simulink model "fw_pos_control"  (R2021a)
settings: Solver=FixedStepAuto  StartTime=0.0  StopTime=5  FixedStep=0.02  RelTol=1e-3
undefined symbols (not defined in the file): DiscIntNeverNeededParam, DT_DEFAULT, FW_AIRSPD_MAX, FW_AIRSPD_MIN, FW_L1_DAMPING, FW_L1_PERIOD, FW_L1_R_SLEW_MAX, FW_R_LIM, FW_T_CLMB_MAX, FW_T_HRATE_FF, FW_T_I_GAIN_PIT, FW_T_I_GAIN_THR, FW_T_PTCH_DAMP, FW_T_RLL2THR, FW_T_SEB_R_FF, FW_T_SINK_MAX, FW_T_SINK_MIN, FW_T_SPD_OMEGA, FW_T_STE_R_TC, FW_T_TAS_TC, FW_T_THR_DAMP, FW_T_VERT_ACC, FW_THR_CRUISE, FW_THR_MAX, FW_THR_MIN, FW_THR_SLEW_MAX, GRAVITY, magnitude
libraries: simulink x28, vrlib x3
(part 1 of 4)
settings Model: DataDictionary=px4_dict.sldd  Creator=DELL  LastModifiedBy=DELL
settings OptimizationCC: DefaultUnderspecifiedDataType=single
settings SFSimCC: SimTargetLang=C++

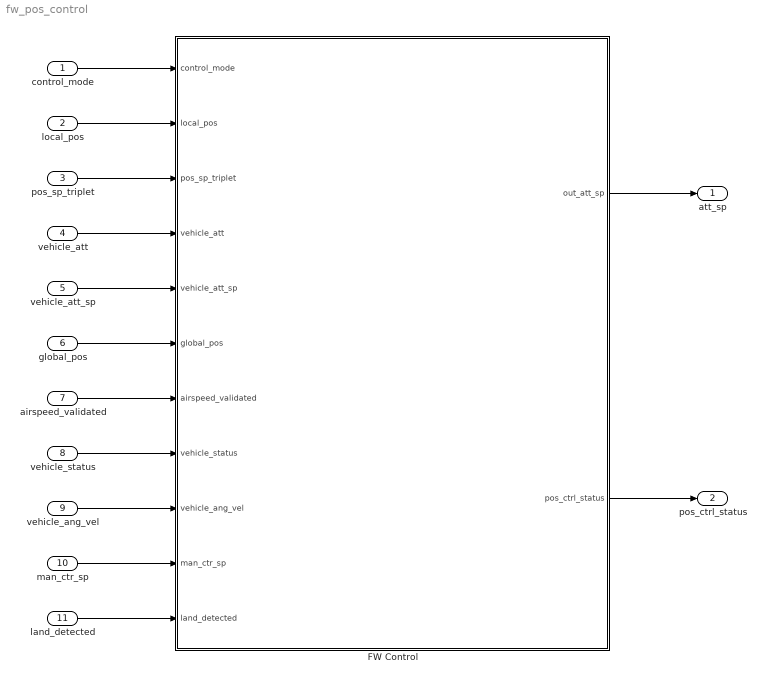
== system fw_pos_control ==
  control_mode : Inport  OutDataTypeStr=Bus: px4_vehicle_control_mode
  local_pos : Inport  Port=2  OutDataTypeStr=Bus: px4_vehicle_local_position
  pos_sp_triplet : Inport  Port=3  OutDataTypeStr=Bus: px4_position_setpoint_triplet
  vehicle_att : Inport  Port=4  OutDataTypeStr=Bus: px4_vehicle_attitude
  vehicle_att_sp : Inport  Port=5  OutDataTypeStr=Bus: px4_vehicle_attitude_setpoint
  global_pos : Inport  Port=6  OutDataTypeStr=Bus: px4_vehicle_global_position
  airspeed_validated : Inport  Port=7  OutDataTypeStr=Bus: px4_airspeed_validated
  vehicle_status : Inport  Port=8  OutDataTypeStr=Bus: px4_vehicle_status
  vehicle_ang_vel : Inport  Port=9  OutDataTypeStr=Bus: px4_vehicle_angular_velocity
  man_ctr_sp : Inport  Port=10  OutDataTypeStr=Bus: px4_manual_control_setpoint
  land_detected : Inport  Port=11  OutDataTypeStr=Bus: px4_vehicle_land_detected
  FW Control : Stateflow chart  TreatAsAtomicUnit=on
  att_sp : Outport
  pos_ctrl_status : Outport  Port=2
  wires:
  airspeed_validated/1 -> FW Control/7(airspeed_validated)
  vehicle_att/1 -> FW Control/4(vehicle_att)
  local_pos/1 -> FW Control/2(local_pos)
  man_ctr_sp/1 -> FW Control/10(man_ctr_sp)
  land_detected/1 -> FW Control/11(land_detected)
  vehicle_status/1 -> FW Control/8(vehicle_status)
  vehicle_att_sp/1 -> FW Control/5(vehicle_att_sp)
  control_mode/1 -> FW Control/1(control_mode)
  FW Control/1(out_att_sp) -> att_sp/1
  vehicle_ang_vel/1 -> FW Control/9(vehicle_ang_vel)
  global_pos/1 -> FW Control/6(global_pos)
  pos_sp_triplet/1 -> FW Control/3(pos_sp_triplet)
  FW Control/2(pos_ctrl_status) -> pos_ctrl_status/1

== system fw_pos_control/FW Control/fixed_wing.position_control.mode_action.l1_navigate_heading ==
  navigation_heading : Inport  OutDataTypeStr=single  PortDimensions=1
  current_heading : Inport  Port=2  OutDataTypeStr=single  PortDimensions=1
  ground_speed_vector : Inport  Port=3  OutDataTypeStr=single  PortDimensions=[1 2]
  att_sp_roll_body : Inport  Port=4  OutDataTypeStr=single  PortDimensions=1
  f : TriggerPort  TriggerType=function-call  VariantControl=(inherit)
      settings: CopyFcn=Stateflow.SLINSF.SimulinkMan.removeBlockPreDeleteFcn  PreDeleteFcn=Stateflow.SLINSF.SimulinkMan.unsafePredeleteFcn
  Constant : Constant  Value=sqrt(2) * pi / FW_L1_PERIOD
      settings: AttributesFormatString=%<Value>
  Constant1 : Constant  Value=false
  Divide : Product  Inputs=*/
  Dot Product1 : DotProduct  InputSameDT=on  OutDataTypeStr=Inherit: Inherit via internal rule
  Gain : Gain  Gain=sqrt(2) * pi / FW_L1_PERIOD
      settings: AttributesFormatString=%<Gain>
  Gain1 : Gain  Gain=2.0
  Product : Product
  Saturation1 : Saturate  UpperLimit=single(pi/2)  LowerLimit=single(-pi/2)
      settings: AttributesFormatString=[%<LowerLimit>,%<UpperLimit>]
  Sin : Trigonometry
  Sqrt1 : Sqrt  SaturateOnIntegerOverflow=on
  Sum : Sum  Inputs=|+-
  Update Roll Setpoint : Subsystem
  wrap -pi~pi : Subsystem
  roll_sp : Outport
  circle_mode : Outport  Port=2
  l1_heading_dis : Outport  Port=3
  wires:
  Constant1/1 -> circle_mode/1
  wrap -pi~pi/1(out) -> Saturation1/1  "eta"
  Sum/1 -> wrap -pi~pi/1(in)
  Saturation1/1 -> Sin/1
  navigation_heading/1 -> Sum/1
  current_heading/1 -> Sum/2
  Dot Product1/1 -> Sqrt1/1
  ground_speed_vector/1 -> Dot Product1/1, Dot Product1/2
  Sqrt1/1 -> Divide/1, Gain/1  "ground_speed_length"
  Product/1 -> Gain1/1
  Sin/1 -> Product/1
  Gain/1 -> Product/2
  Constant/1 -> Divide/2  "heading_omega"
  Divide/1 -> l1_heading_dis/1
  att_sp_roll_body/1 -> Update Roll Setpoint/1(att_sp_roll_body1)
  Gain1/1 -> Update Roll Setpoint/2(lateral_accel)
  Update Roll Setpoint/1(roll_new) -> roll_sp/1

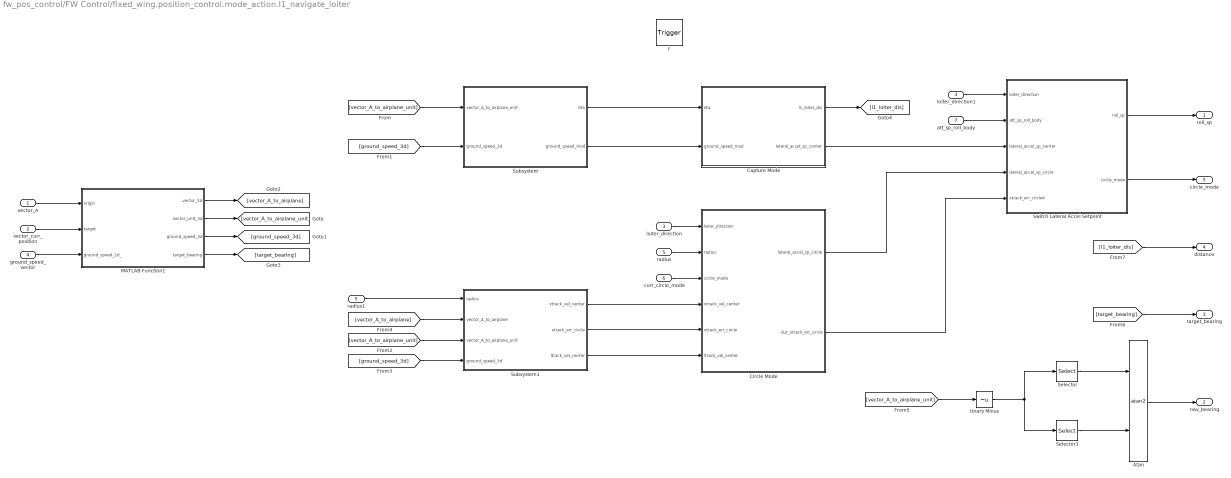
== system fw_pos_control/FW Control/fixed_wing.position_control.mode_action.l1_navigate_loiter ==
  vector_A : Inport  OutDataTypeStr=double  PortDimensions=[1 2]
  vector_curr_position : Inport  Port=2  OutDataTypeStr=double  PortDimensions=[1 2]
  loiter_direction : Inport  Port=3  OutDataTypeStr=int8  PortDimensions=1
  ground_speed_vector : Inport  Port=4  OutDataTypeStr=single  PortDimensions=[1 2]
  radius : Inport  Port=5  OutDataTypeStr=single  PortDimensions=1
  curr_circle_mode : Inport  Port=6  OutDataTypeStr=boolean  PortDimensions=1
  att_sp_roll_body : Inport  Port=7  OutDataTypeStr=single  PortDimensions=1
  f : TriggerPort  TriggerType=function-call  VariantControl=(inherit)
      settings: CopyFcn=Stateflow.SLINSF.SimulinkMan.removeBlockPreDeleteFcn  PreDeleteFcn=Stateflow.SLINSF.SimulinkMan.unsafePredeleteFcn
  Atan : Trigonometry  Operator=atan2
  Capture Mode : Subsystem
  Circle Mode : Subsystem
  MATLAB Function1 : MATLAB Function  TreatAsAtomicUnit=on
  Selector : Selector  InputPortWidth=3  IndexOptions=Index vector (dialog)  Indices=[2]  OutputSizes=1
  Selector1 : Selector  InputPortWidth=3  IndexOptions=Index vector (dialog)  Indices=[1]  OutputSizes=1
  Subsystem : Subsystem
  Subsystem1 : Subsystem
  Switch Lateral Accel Setpoint : Subsystem
  Unary Minus : UnaryMinus
  loiter_direction1 : InportShadow  Port=3  OutDataTypeStr=int8  PortDimensions=1
  radius1 : InportShadow  Port=5  OutDataTypeStr=single  PortDimensions=1
  roll_sp : Outport
  nav_bearing : Outport  Port=2
  target_bearing : Outport  Port=3
  distance : Outport  Port=4
  circle_mode : Outport  Port=5
  wires:
  vector_curr_position/1 -> MATLAB Function1/2(target)
  vector_A/1 -> MATLAB Function1/1(origin)
  ground_speed_vector/1 -> MATLAB Function1/3(ground_speed_2d_)
  Subsystem/1(eta) -> Capture Mode/1(eta)
  Capture Mode/2(lateral_accel_sp_center) -> Switch Lateral Accel Setpoint/3(lateral_accel_sp_center)
  Capture Mode/1(l1_loiter_dis) -> [l1_loiter_dis]
  Subsystem/2(ground_speed_mod) -> Capture Mode/2(ground_speed_mod)
  loiter_direction/1 -> Circle Mode/1(loiter_direction)
  radius/1 -> Circle Mode/2(radius)
  Circle Mode/1(lateral_accel_sp_circle) -> Switch Lateral Accel Setpoint/4(lateral_accel_sp_circle)
  Subsystem1/2(xtrack_err_circle) -> Circle Mode/5(xtrack_err_circle)
  Subsystem1/1(xtrack_vel_center) -> Circle Mode/4(xtrack_vel_center)
  MATLAB Function1/2(vector_unit_3d) -> [vector_A_to_airplane_unit]
  MATLAB Function1/3(ground_speed_3d) -> [ground_speed_3d]
  [vector_A_to_airplane_unit] -> Subsystem/1(vector_A_to_airplane_unit)
  [ground_speed_3d] -> Subsystem/2(ground_speed_3d)
  [ground_speed_3d] -> Subsystem1/4(ground_speed_3d)
  radius1/1 -> Subsystem1/1(radius)
  MATLAB Function1/1(vector_3d) -> [vector_A_to_airplane]
  [vector_A_to_airplane_unit] -> Subsystem1/3(vector_A_to_airplane_unit)
  [vector_A_to_airplane] -> Subsystem1/2(vector_A_to_airplane)
  Subsystem1/3(ltrack_vel_center) -> Circle Mode/6(ltrack_vel_center)
  curr_circle_mode/1 -> Circle Mode/3(circle_mode)
  Circle Mode/2(out_xtrack_err_circle) -> Switch Lateral Accel Setpoint/5(xtrack_err_circle4)
  loiter_direction1/1 -> Switch Lateral Accel Setpoint/1(loiter_direction)
  Switch Lateral Accel Setpoint/2(circle_mode) -> circle_mode/1
  [vector_A_to_airplane_unit] -> Unary Minus/1
  Selector1/1 -> Atan/2
  Selector/1 -> Atan/1
  Unary Minus/1 -> Selector1/1, Selector/1
  Atan/1 -> nav_bearing/1
  Switch Lateral Accel Setpoint/1(roll_sp) -> roll_sp/1
  att_sp_roll_body/1 -> Switch Lateral Accel Setpoint/2(att_sp_roll_body)
  MATLAB Function1/4(target_bearing) -> [target_bearing]
  [l1_loiter_dis] -> distance/1
  [target_bearing] -> target_bearing/1

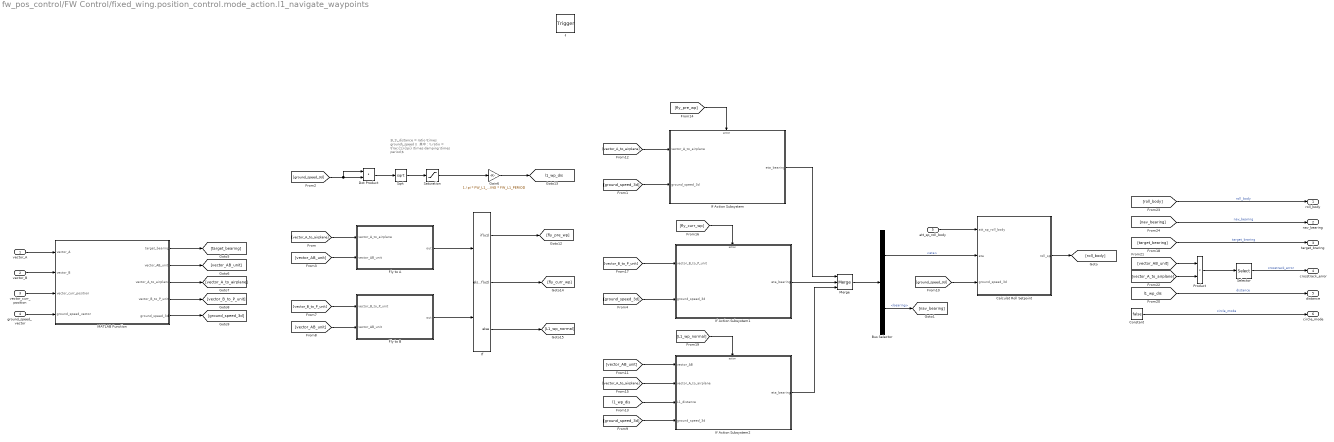
== system fw_pos_control/FW Control/fixed_wing.position_control.mode_action.l1_navigate_waypoints ==
  note: $L1\_distance = ratio \times ground\_speed \\ 其中：\\ ratio = \frac{1}{\pi} \times damping \times period;$
  vector_A : Inport  OutDataTypeStr=double  PortDimensions=[1 2]
  vector_B : Inport  Port=2  OutDataTypeStr=double  PortDimensions=[1 2]
  vector_curr_position : Inport  Port=3  OutDataTypeStr=double  PortDimensions=[1 2]
  ground_speed_vector : Inport  Port=4  OutDataTypeStr=single  PortDimensions=[1 2]
  att_sp_roll_body : Inport  Port=5  OutDataTypeStr=single  PortDimensions=1
  f : TriggerPort  TriggerType=function-call  VariantControl=(inherit)
      settings: CopyFcn=Stateflow.SLINSF.SimulinkMan.removeBlockPreDeleteFcn  PreDeleteFcn=Stateflow.SLINSF.SimulinkMan.unsafePredeleteFcn
  Bus Selector : BusSelector  OutputSignals=eta,bearing
  Calculat Roll Setpoint : Subsystem
  Constant : Constant  Value=false
  Dot Product : DotProduct  InputSameDT=on  OutDataTypeStr=Inherit: Inherit via internal rule
  Fly to A : Subsystem
  Fly to B : Subsystem
  Gain6 : Gain  Gain=1 / pi * FW_L1_DAMPING * FW_L1_PERIOD
      settings: AttributesFormatString=%<Gain>
  If : If  NumInputs=2  IfExpression=u1  ElseIfExpressions=u2
  If Action Subsystem : Subsystem  TreatAsAtomicUnit=on
  If Action Subsystem1 : Subsystem  TreatAsAtomicUnit=on
  If Action Subsystem2 : Subsystem  TreatAsAtomicUnit=on
  MATLAB Function : MATLAB Function  TreatAsAtomicUnit=on
  Merge : Merge  Inputs=3
  Product : Product
  Saturation : Saturate  UpperLimit=single(inf)  LowerLimit=single(0.1)
      settings: AttributesFormatString=[%<LowerLimit>,%<UpperLimit>]
  Selector : Selector  InputPortWidth=3  IndexOptions=Index vector (dialog)  Indices=[3]  OutputSizes=1
  Sqrt : Sqrt  SaturateOnIntegerOverflow=on
  roll_body : Outport
  nav_bearing : Outport  Port=2
  target_braring : Outport  Port=3
  crosstrack_error : Outport  Port=4
  distance : Outport  Port=5
  circle_mode : Outport  Port=6
  tag scope: l1_wp_dis=global
  wires:
  MATLAB Function/4(vector_B_to_P_unit) -> [vector_B_to_P_unit]
  MATLAB Function/2(vector_AB_unit) -> [vector_AB_unit]
  vector_curr_position/1 -> MATLAB Function/3(vector_curr_position)
  vector_A/1 -> MATLAB Function/1(vector_A)
  MATLAB Function/1(target_bearing) -> [target_bearing]
  vector_B/1 -> MATLAB Function/2(vector_B)
  MATLAB Function/3(vector_A_to_airplane) -> [vector_A_to_airplane]
  ground_speed_vector/1 -> MATLAB Function/4(ground_speed_vector)
  MATLAB Function/5(ground_speed_3d) -> [ground_speed_3d]
  [vector_A_to_airplane] -> Fly to A/1(vector_A_to_airplane)
  [vector_AB_unit] -> Fly to B/2(vector_AB_unit)
  [vector_B_to_P_unit] -> Fly to B/1(vector_B_to_P_unit)
  [vector_AB_unit] -> Fly to A/2(vector_AB_unit)
  Dot Product/1 -> Sqrt/1
  Sqrt/1 -> Saturation/1
  Saturation/1 -> Gain6/1
  [ground_speed_3d] -> Dot Product/1, Dot Product/2
  Gain6/1 -> [l1_wp_dis]
  If/1 -> [fly_pre_wp]
  Fly to A/1(out) -> If/1
  [l1_wp_dis] -> distance/1  "distance"
  [fly_pre_wp] -> If Action Subsystem/Action
  [ground_speed_3d] -> If Action Subsystem2/4(ground_speed_3d)
  [vector_AB_unit] -> If Action Subsystem2/1(vector_AB)
  [L1_wp_normal] -> If Action Subsystem2/Action
  If/2 -> [fly_curr_wp]
  [l1_wp_dis] -> If Action Subsystem2/3(L1_distance)
  [vector_A_to_airplane] -> If Action Subsystem2/2(vector_A_to_airplane)
  [fly_curr_wp] -> If Action Subsystem1/Action
  [vector_B_to_P_unit] -> If Action Subsystem1/1(vector_B_to_P_unit)
  [vector_A_to_airplane] -> If Action Subsystem/1(vector_A_to_airplane)
  [ground_speed_3d] -> If Action Subsystem/2(ground_speed_3d)
  If/3 -> [L1_wp_normal]
  [ground_speed_3d] -> If Action Subsystem1/2(ground_speed_3d)
  If Action Subsystem/1(eta_bearing) -> Merge/1
  Fly to B/1(out) -> If/2
  [ground_speed_3d] -> Calculat Roll Setpoint/3(ground_speed_3d)
  att_sp_roll_body/1 -> Calculat Roll Setpoint/1(att_sp_roll_body)
  If Action Subsystem1/1(eta_bearing) -> Merge/2
  Merge/1 -> Bus Selector/1
  Bus Selector/1 -> Calculat Roll Setpoint/2(eta)  "<eta>"
  If Action Subsystem2/1(eta_bearing) -> Merge/3
  Constant/1 -> circle_mode/1  "circle_mode"
  [target_bearing] -> target_braring/1  "target_braring"
  [vector_A_to_airplane] -> Product/2
  [vector_AB_unit] -> Product/1
  Bus Selector/2 -> [nav_bearing]  "<bearing>"
  [nav_bearing] -> nav_bearing/1  "nav_bearing"
  Product/1 -> Selector/1
  Selector/1 -> crosstrack_error/1  "crosstrack_error"
  Calculat Roll Setpoint/1(roll_sp) -> [roll_body]
  [roll_body] -> roll_body/1  "roll_body"

== system fw_pos_control/FW Control/fixed_wing.position_control.mode_action.tecs_controller ==
  tecs_input : Inport  OutDataTypeStr=Bus: px4_tecs_input  PortDimensions=1
  f : TriggerPort  TriggerType=function-call  VariantControl=(inherit)
      settings: CopyFcn=Stateflow.SLINSF.SimulinkMan.removeBlockPreDeleteFcn  PreDeleteFcn=Stateflow.SLINSF.SimulinkMan.unsafePredeleteFcn
  Tecs Logical : Stateflow chart  TreatAsAtomicUnit=on
  Update Energy Estimates : Subsystem
  Update Height State and Height Setpoint State : Subsystem
  Update Speed State and Speed Setpoint State : Subsystem
  Update Throttle Setpoint and Pitch Setpoint : Subsystem
  tecs_input2 : InportShadow  OutDataTypeStr=Bus: px4_tecs_input  PortDimensions=1
  tecs_input3 : InportShadow  OutDataTypeStr=Bus: px4_tecs_input  PortDimensions=1
  tecs_input4 : InportShadow  OutDataTypeStr=Bus: px4_tecs_input  PortDimensions=1
  throttle_sp : Outport
  pitch_sp : Outport  Port=2
  hgt_rate_sp : Outport  Port=3
  tecs_mode : Outport  Port=4
  tag scope: SKE_weighting=global, SPE_weighting=global, un_des_rec=global, un_spd_det=global
  wires:
  Update Throttle Setpoint and Pitch Setpoint/2(pitch_sp) -> pitch_sp/1
  tecs_input/1 -> Update Speed State and Speed Setpoint State/1(tecs), Update Height State and Height Setpoint State/1(tecs)
  Update Speed State and Speed Setpoint State/1(tas_state) -> Update Energy Estimates/2(tas_state)
  Update Speed State and Speed Setpoint State/2(tas_sp_state) -> Update Energy Estimates/3(tas_sp_state)
  Update Height State and Height Setpoint State/1(hgt_state) -> Update Energy Estimates/4(hgt_state)
  Update Height State and Height Setpoint State/2(hgt_sp_state) -> Update Energy Estimates/5(hgt_sp_state)
  Update Energy Estimates/4(SEB_rate_error) -> Update Throttle Setpoint and Pitch Setpoint/5(SEB_rate_error)
  Update Energy Estimates/3(SEB_rate_sp) -> Update Throttle Setpoint and Pitch Setpoint/4(SEB_rate_sp)
  Tecs Logical/1(underspeed_detected) -> [un_spd_det]
  Tecs Logical/2(uncommanded_descent_recovery) -> [un_des_rec]
  tecs_input4/1 -> Tecs Logical/1(tecs)
  [last_thr_sp] -> Tecs Logical/2(last_throttle_setpoint)
  [tas] -> Tecs Logical/3(tas)
  Tecs Logical/4(SKE_weighting_) -> [SKE_weighting]
  Tecs Logical/3(SPE_weighting_) -> [SPE_weighting]
  [STE_rate] -> Tecs Logical/4(STE_rate)
  [STE_error] -> Tecs Logical/5(STE_error)
  tecs_input2/1 -> Update Throttle Setpoint and Pitch Setpoint/1(tecs)
  Update Energy Estimates/1(STE_rate_sp) -> Update Throttle Setpoint and Pitch Setpoint/2(STE_rate_error)
  Update Energy Estimates/2(STE_rate_error) -> Update Throttle Setpoint and Pitch Setpoint/3(STE_rate_sp)
  Update Throttle Setpoint and Pitch Setpoint/1(throttle_sp) -> throttle_sp/1
  Tecs Logical/5(tecs_mode) -> tecs_mode/1
  tecs_input3/1 -> Update Energy Estimates/1(tecs)
  Update Energy Estimates/5(hgt_rate_sp) -> hgt_rate_sp/1

== system fw_pos_control/FW Control/fixed_wing.position_control.mode_action.l1_navigate_heading/Update Roll Setpoint ==
  att_sp_roll_body1 : Inport  PortDimensions=1
  lateral_accel : Inport  Port=2
  Compare To Zero : simulink/Logic and Bit Operations/Compare To Zero  relop=>  OutDataTypeStr=boolean
  Constant2 : Constant  Value=FW_L1_R_SLEW_MAX
      settings: AttributesFormatString=%<Value>
  Constant3 : Constant  Value=FW_L1_R_SLEW_MAX
      settings: AttributesFormatString=%<Value>
  Gain2 : Gain  Gain=1.0 / GRAVITY
      settings: AttributesFormatString=%<Gain>
  IsFinite1 : RelationalOperator  Operator=isFinite  OutDataTypeStr=boolean  RndMeth=Simplest
  Saturation : Saturate  UpperLimit=FW_R_LIM  LowerLimit=-FW_R_LIM
      settings: AttributesFormatString=[%<LowerLimit>,%<UpperLimit>]
  Saturation Dynamic : simulink/Discontinuities/Saturation Dynamic  OutMin=[]  OutMax=[]  OutDataTypeStr=Inherit: Same as second input  OutDataType=fixdt(1, 16)  OutScaling=2^-10  DoSatur=off
  Sum1 : Sum  Inputs=|++
  Sum2 : Sum  Inputs=-+|
  Switch1 : Switch  Criteria=u2 > Threshold
  Switch2 : Switch  Criteria=u2 > Threshold
  Weighted Sample Time : SampleTimeMath  TsampMathOp=*
  att_sp_roll_body1_1 : InportShadow  PortDimensions=1
  att_sp_roll_body1_2 : InportShadow  PortDimensions=1
  roll_new : Outport
  wires:
  Saturation Dynamic/1 -> Switch1/1
  Sum2/1 -> Saturation Dynamic/3
  att_sp_roll_body1/1 -> Sum1/1
  Constant2/1 -> Weighted Sample Time/1
  IsFinite1/1 -> Switch2/2
  Weighted Sample Time/1 -> Sum1/2, Sum2/1
  att_sp_roll_body1_1/1 -> Sum2/2
  att_sp_roll_body1_2/1 -> Switch2/3
  lateral_accel/1 -> Gain2/1
  Sum1/1 -> Saturation Dynamic/1
  Gain2/1 -> Saturation/1
  Constant3/1 -> Compare To Zero/1
  Compare To Zero/1 -> Switch1/2
  Saturation/1 -> IsFinite1/1, Switch2/1, Saturation Dynamic/2  "roll_new"
  Switch2/1 -> Switch1/3
  Switch1/1 -> roll_new/1

== system fw_pos_control/FW Control/fixed_wing.position_control.mode_action.l1_navigate_heading/wrap -pi~pi ==
  in : Inport
  Constant1 : Constant  Value=2*pi  OutDataTypeStr=single
  Mod : Math  Operator=mod  SaturateOnIntegerOverflow=on
  Sum1 : Sum  Inputs=|+-
  Switch : Switch  Criteria=u2 > Threshold  Threshold=pi
  out : Outport
  wires:
  Sum1/1 -> Switch/1
  Mod/1 -> Switch/3, Switch/2, Sum1/1
  Constant1/1 -> Sum1/2, Mod/2
  Switch/1 -> out/1
  in/1 -> Mod/1

== system fw_pos_control/FW Control/fixed_wing.position_control.mode_action.l1_navigate_loiter/Capture Mode ==
  note: $lateral\_accel\_sp\_center = \frac{K\_L1 \times ground\_speed^{2}}{L1\_distance \times sin(\eta);} \\ 其中：\\ L1\_distance = L1\_ratio \times ground\_speed;$
  eta : Inport
  ground_speed_mod : Inport  Port=2
  Divide1 : Product  Inputs=*/
  Gain : Gain  Gain=4 * FW_L1_DAMPING^2
      settings: AttributesFormatString=%<Gain>
  Gain1 : Gain  Gain=1 / pi * FW_L1_DAMPING * FW_L1_PERIOD
      settings: AttributesFormatString=%<Gain>
  Math Function2 : Math  Operator=magnitude^2  SaturateOnIntegerOverflow=on
  Product1 : Product
  Sin1 : Trigonometry
  ground_speed_mod1 : InportShadow  Port=2
  l1_loiter_dis : Outport
  lateral_accel_sp_center : Outport  Port=2
  wires:
  Gain/1 -> Divide1/1
  Sin1/1 -> Product1/2
  Divide1/1 -> lateral_accel_sp_center/1
  Math Function2/1 -> Gain/1
  Gain1/1 -> l1_loiter_dis/1, Product1/1  "L1_distance"
  Product1/1 -> Divide1/2
  eta/1 -> Sin1/1
  ground_speed_mod/1 -> Math Function2/1
  ground_speed_mod1/1 -> Gain1/1

== system fw_pos_control/FW Control/fixed_wing.position_control.mode_action.l1_navigate_loiter/Circle Mode ==
  loiter_direction : Inport
  radius : Inport  Port=2
  circle_mode : Inport  Port=3
  xtrack_vel_center : Inport  Port=4
  xtrack_err_circle : Inport  Port=5
  ltrack_vel_center : Inport  Port=6
  Divide2 : Product  Inputs=*/
  Gain4 : Gain  Gain=0.5
  Magnitude Squared : Math  Operator=magnitude^2  SaturateOnIntegerOverflow=on
  Max : MinMax  Function=max  Inputs=2
  PD Terms : Subsystem
  Product2 : Product
  Product3 : Product
  Sum2 : Sum  Inputs=++|
  Sum3 : Sum  Inputs=|++
  loiter_direction1 : InportShadow
  xtrack_err_circle1 : InportShadow  Port=5
  xtrack_err_circle2 : InportShadow  Port=5
  lateral_accel_sp_circle : Outport
  out_xtrack_err_circle : Outport  Port=2
  tag scope: tangent_vel=global
  wires:
  PD Terms/1(lateral_accel_sp_circle_pd) -> Sum3/2
  Gain4/1 -> Max/1
  Product2/1 -> [tangent_vel], Magnitude Squared/1
  radius/1 -> Sum2/1, Gain4/1
  Sum3/1 -> Product3/1
  Divide2/1 -> Sum3/1  "lateral_accel_sp_circle_centripetal"
  Sum2/1 -> Max/2
  Magnitude Squared/1 -> Divide2/1
  Max/1 -> Divide2/2
  loiter_direction1/1 -> Product3/2
  Product3/1 -> lateral_accel_sp_circle/1
  xtrack_vel_center/1 -> Product2/1
  loiter_direction/1 -> Product2/2
  ltrack_vel_center/1 -> PD Terms/2(xtrack_vel_circle)
  xtrack_err_circle/1 -> Sum2/2
  xtrack_err_circle1/1 -> PD Terms/1(xtrack_err_circle)
  circle_mode/1 -> PD Terms/3(circle_mode)
  xtrack_err_circle2/1 -> out_xtrack_err_circle/1

== system fw_pos_control/FW Control/fixed_wing.position_control.mode_action.l1_navigate_loiter/Subsystem ==
  note: $\begin{cases} a \times b &= \left | a \right | {\left | b \right | \sin\theta \\ a \cdot b &= \left | a \right | {\left | b \right | \cos\theta \end{cases} \\ \quad \tan{\theta} = \frac{a \times b}{a \cdot b}$
  vector_A_to_airplane_unit : Inport
  ground_speed_3d : Inport  Port=2
  Atan2 : Trigonometry  Operator=atan2
  Cross Product : vrlib/Utilities/Cross Product
  Dot Product : DotProduct  InputSameDT=on  OutDataTypeStr=Inherit: Inherit via internal rule
  Dot Product1 : DotProduct  InputSameDT=on  OutDataTypeStr=Inherit: Inherit via internal rule
  Saturation : Saturate  UpperLimit=single(inf)  LowerLimit=single(0.1)
      settings: AttributesFormatString=[%<LowerLimit>,%<UpperLimit>]
  Saturation2 : Saturate  UpperLimit=single(pi/2)  LowerLimit=single(-pi/2)
      settings: AttributesFormatString=[%<LowerLimit>,%<UpperLimit>]
  Selector : Selector  InputPortWidth=3  IndexOptions=Index vector (dialog)  Indices=[3]  OutputSizes=1
  Sqrt : Sqrt  SaturateOnIntegerOverflow=on
  Unary Minus : UnaryMinus
  ground_speed_3d1 : InportShadow  Port=2
  ground_speed_3d2 : InportShadow  Port=2
  vector_A_to_airplane_unit1 : InportShadow
  eta : Outport
  ground_speed_mod : Outport  Port=2
  wires:
  Cross Product/1 -> Selector/1
  Dot Product1/1 -> Unary Minus/1
  vector_A_to_airplane_unit/1 -> Cross Product/1
  Atan2/1 -> Saturation2/1
  Selector/1 -> Atan2/1
  Unary Minus/1 -> Atan2/2
  Saturation2/1 -> eta/1
  ground_speed_3d/1 -> Cross Product/2
  ground_speed_3d1/1 -> Dot Product1/2
  vector_A_to_airplane_unit1/1 -> Dot Product1/1
  ground_speed_3d2/1 -> Dot Product/1, Dot Product/2
  Sqrt/1 -> Saturation/1
  Dot Product/1 -> Sqrt/1
  Saturation/1 -> ground_speed_mod/1

== system fw_pos_control/FW Control/fixed_wing.position_control.mode_action.l1_navigate_loiter/Subsystem1 ==
  radius : Inport
  vector_A_to_airplane : Inport  Port=2
  vector_A_to_airplane_unit : Inport  Port=3
  ground_speed_3d : Inport  Port=4
  Cross Product : vrlib/Utilities/Cross Product
  Dot Product1 : DotProduct  InputSameDT=on  OutDataTypeStr=Inherit: Inherit via internal rule
  Dot Product2 : DotProduct  InputSameDT=on  OutDataTypeStr=Inherit: Inherit via internal rule
  Selector : Selector  InputPortWidth=3  IndexOptions=Index vector (dialog)  Indices=[3]  OutputSizes=1
  Sqrt1 : Sqrt  SaturateOnIntegerOverflow=on
  Sum : Sum  Inputs=|+-
  Unary Minus : UnaryMinus
  ground_speed_3d2 : InportShadow  Port=4
  vector_A_to_airplane_unit2 : InportShadow  Port=3
  xtrack_vel_center : Outport
  xtrack_err_circle : Outport  Port=2
  ltrack_vel_center : Outport  Port=3
  wires:
  vector_A_to_airplane/1 -> Dot Product2/2, Dot Product2/1
  Dot Product2/1 -> Sqrt1/1
  ground_speed_3d/1 -> Cross Product/2
  Selector/1 -> xtrack_vel_center/1
  vector_A_to_airplane_unit/1 -> Cross Product/1
  Cross Product/1 -> Selector/1
  Sqrt1/1 -> Sum/1
  Sum/1 -> xtrack_err_circle/1
  radius/1 -> Sum/2
  Dot Product1/1 -> Unary Minus/1
  ground_speed_3d2/1 -> Dot Product1/2
  Unary Minus/1 -> ltrack_vel_center/1
  vector_A_to_airplane_unit2/1 -> Dot Product1/1

== system fw_pos_control/FW Control/fixed_wing.position_control.mode_action.l1_navigate_loiter/Switch Lateral Accel Setpoint ==
  note: Switch between circle (loiter) and capture (towards waypoint center) mode when the commands switch over. Only fly towards waypoint if outside the circle.
  loiter_direction : Inport
  att_sp_roll_body : Inport  Port=2  PortDimensions=1
  lateral_accel_sp_center : Inport  Port=3
  lateral_accel_sp_circle : Inport  Port=4
  xtrack_err_circle4 : Inport  Port=5
  AND1 : Logic  IconShape=distinctive  AllPortsSameDT=off  OutDataTypeStr=boolean
  Compare To Zero1 : simulink/Logic and Bit Operations/Compare To Zero  relop=<  OutDataTypeStr=boolean
  Compare To Zero3 : simulink/Logic and Bit Operations/Compare To Zero  relop=>  OutDataTypeStr=boolean
  If Action Subsystem : Subsystem  TreatAsAtomicUnit=on
  If Action Subsystem1 : Subsystem  TreatAsAtomicUnit=on
  If1 : If  IfExpression=u1
  Merge : Merge
  Merge1 : Merge
  Product : Product
  Sum5 : Sum  Inputs=|+-
  Update Roll Setpoint : Subsystem
  lateral_accel_sp_center1 : InportShadow  Port=3
  lateral_accel_sp_circle1 : InportShadow  Port=4
  roll_sp : Outport
  circle_mode : Outport  Port=2
  wires:
  If1/2 -> If Action Subsystem1/Action
  xtrack_err_circle4/1 -> Compare To Zero3/1
  If1/1 -> If Action Subsystem/Action
  AND1/1 -> If1/1
  Product/1 -> Compare To Zero1/1
  Compare To Zero1/1 -> AND1/1
  Compare To Zero3/1 -> AND1/2  "飞机在圆外"
  lateral_accel_sp_center/1 -> Sum5/1
  lateral_accel_sp_circle/1 -> Sum5/2
  lateral_accel_sp_center1/1 -> If Action Subsystem/1(lateral_accel_sp_center)
  lateral_accel_sp_circle1/1 -> If Action Subsystem1/1(lateral_accel_sp_circle1)
  Merge1/1 -> circle_mode/1
  Sum5/1 -> Product/2
  loiter_direction/1 -> Product/1
  If Action Subsystem1/2(circle_mode) -> Merge1/2
  If Action Subsystem/1(circle_mode) -> Merge1/1
  If Action Subsystem1/1(lateral_accel_sp) -> Merge/2
  If Action Subsystem/2(lateral_accel_sp) -> Merge/1
  att_sp_roll_body/1 -> Update Roll Setpoint/1(att_sp_roll_body)
  Merge/1 -> Update Roll Setpoint/2(lateral_accel)  "lateral_accel"
  Update Roll Setpoint/1(roll_sp) -> roll_sp/1

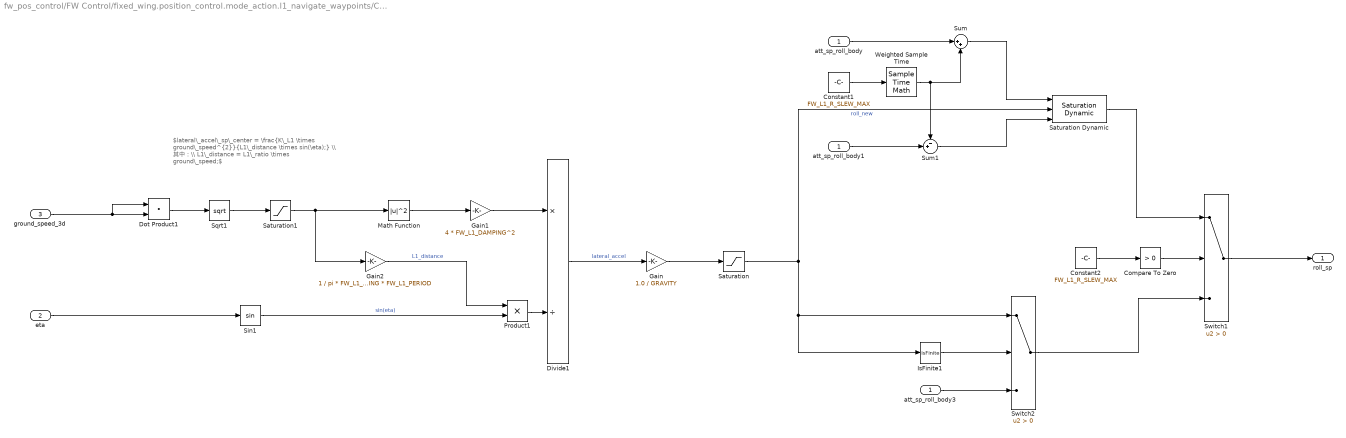
== system fw_pos_control/FW Control/fixed_wing.position_control.mode_action.l1_navigate_waypoints/Calculat Roll Setpoint ==
  note: $lateral\_accel\_sp\_center = \frac{K\_L1 \times ground\_speed^{2}}{L1\_distance \times sin(\eta);} \\ 其中：\\ L1\_distance = L1\_ratio \times ground\_speed;$
  att_sp_roll_body : Inport  PortDimensions=1
  eta : Inport  Port=2
  ground_speed_3d : Inport  Port=3
  Compare To Zero : simulink/Logic and Bit Operations/Compare To Zero  relop=>  OutDataTypeStr=boolean
  Constant1 : Constant  Value=FW_L1_R_SLEW_MAX
      settings: AttributesFormatString=%<Value>
  Constant2 : Constant  Value=FW_L1_R_SLEW_MAX
      settings: AttributesFormatString=%<Value>
  Divide1 : Product  Inputs=*/
  Dot Product1 : DotProduct  InputSameDT=on  OutDataTypeStr=Inherit: Inherit via internal rule
  Gain : Gain  Gain=1.0 / GRAVITY
      settings: AttributesFormatString=%<Gain>
  Gain1 : Gain  Gain=4 * FW_L1_DAMPING^2
      settings: AttributesFormatString=%<Gain>
  Gain2 : Gain  Gain=1 / pi * FW_L1_DAMPING * FW_L1_PERIOD
      settings: AttributesFormatString=%<Gain>
  IsFinite1 : RelationalOperator  Operator=isFinite  OutDataTypeStr=boolean  RndMeth=Simplest
  Math Function : Math  Operator=magnitude^2  SaturateOnIntegerOverflow=on
  Product1 : Product
  Saturation : Saturate  UpperLimit=FW_R_LIM  LowerLimit=-FW_R_LIM
      settings: AttributesFormatString=[%<LowerLimit>,%<UpperLimit>]
  Saturation Dynamic : simulink/Discontinuities/Saturation Dynamic  OutMin=[]  OutMax=[]  OutDataTypeStr=Inherit: Same as second input  OutDataType=fixdt(1, 16)  OutScaling=2^-10  DoSatur=off
  Saturation1 : Saturate  UpperLimit=single(inf)  LowerLimit=single(0.1)
      settings: AttributesFormatString=[%<LowerLimit>,%<UpperLimit>]
  Sin1 : Trigonometry
  Sqrt1 : Sqrt  SaturateOnIntegerOverflow=on
  Sum : Sum  Inputs=|++
  Sum1 : Sum  Inputs=-+|
  Switch1 : Switch  Criteria=u2 > Threshold
  Switch2 : Switch  Criteria=u2 > Threshold
  Weighted Sample Time : SampleTimeMath  TsampMathOp=*
  att_sp_roll_body1 : InportShadow  PortDimensions=1
  att_sp_roll_body3 : InportShadow  PortDimensions=1
  roll_sp : Outport
  wires:
  Product1/1 -> Divide1/2
  Sin1/1 -> Product1/2  "sin(eta)"
  Gain2/1 -> Product1/1  "L1_distance"
  Saturation1/1 -> Gain2/1, Math Function/1
  Gain1/1 -> Divide1/1
  eta/1 -> Sin1/1
  Math Function/1 -> Gain1/1
  Sqrt1/1 -> Saturation1/1
  ground_speed_3d/1 -> Dot Product1/2, Dot Product1/1
  Dot Product1/1 -> Sqrt1/1
  Sum1/1 -> Saturation Dynamic/3
  Weighted Sample Time/1 -> Sum/2, Sum1/1
  Divide1/1 -> Gain/1  "lateral_accel"
  Sum/1 -> Saturation Dynamic/1
  att_sp_roll_body/1 -> Sum/1
  Constant1/1 -> Weighted Sample Time/1
  Gain/1 -> Saturation/1
  Saturation Dynamic/1 -> Switch1/1
  Saturation/1 -> IsFinite1/1, Switch2/1, Saturation Dynamic/2  "roll_new"
  att_sp_roll_body1/1 -> Sum1/2
  Constant2/1 -> Compare To Zero/1
  Compare To Zero/1 -> Switch1/2
  Switch1/1 -> roll_sp/1
  IsFinite1/1 -> Switch2/2
  att_sp_roll_body3/1 -> Switch2/3
  Switch2/1 -> Switch1/3

== system fw_pos_control/FW Control/fixed_wing.position_control.mode_action.l1_navigate_waypoints/Fly to A ==
  vector_A_to_airplane : Inport
  vector_AB_unit : Inport  Port=2
  AND : Logic  IconShape=distinctive  AllPortsSameDT=off  OutDataTypeStr=boolean
  Compare To Constant : simulink/Logic and Bit Operations/Compare To Constant  relop=<  const=single(-0.7071)  OutDataTypeStr=boolean
      settings: AttributesFormatString=%<const>
  Compare To Zero : simulink/Logic and Bit Operations/Compare To Zero  relop=>  OutDataTypeStr=boolean
  Divide : Product  Inputs=*/
  Dot Product1 : DotProduct  InputSameDT=on  OutDataTypeStr=Inherit: Inherit via internal rule
  Dot Product4 : DotProduct  InputSameDT=on  OutDataTypeStr=Inherit: Inherit via internal rule
  Saturation1 : Saturate  UpperLimit=inf  LowerLimit=1
      settings: AttributesFormatString=[%<LowerLimit>,%<UpperLimit>]
  Sqrt2 : Sqrt  SaturateOnIntegerOverflow=on
  Sum : Sum  Inputs=|+-
  vector_A_to_airplane1 : InportShadow
  out : Outport
  wires:
  Dot Product1/1 -> Divide/1  "alongTrackDist"
  Saturation1/1 -> Divide/2
  Sum/1 -> Compare To Zero/1
  Divide/1 -> Compare To Constant/1
  Compare To Zero/1 -> AND/1
  vector_AB_unit/1 -> Dot Product1/2
  Dot Product4/1 -> Sqrt2/1
  Sqrt2/1 -> Sum/1, Saturation1/1  "distance_A_to_airplane"
  Compare To Constant/1 -> AND/2
  vector_A_to_airplane/1 -> Dot Product4/1, Dot Product4/2
  vector_A_to_airplane1/1 -> Dot Product1/1
  AND/1 -> out/1
  [l1_wp_dis] -> Sum/2

== system fw_pos_control/FW Control/fixed_wing.position_control.mode_action.l1_navigate_waypoints/Fly to B ==
  vector_B_to_P_unit : Inport
  vector_AB_unit : Inport  Port=2
  Abs : Abs
  Atan2 : Trigonometry  Operator=atan2
  Compare To Constant1 : simulink/Logic and Bit Operations/Compare To Constant  relop=<  const=single(100*pi/180)  OutDataTypeStr=boolean
      settings: AttributesFormatString=%<const>
  Cross Product : vrlib/Utilities/Cross Product
  Dot Product3 : DotProduct  InputSameDT=on  OutDataTypeStr=Inherit: Inherit via internal rule
  Selector : Selector  InputPortWidth=3  IndexOptions=Index vector (dialog)  Indices=[3]  OutputSizes=1
  out : Outport
  wires:
  Abs/1 -> Compare To Constant1/1
  Cross Product/1 -> Selector/1
  Selector/1 -> Atan2/1
  Dot Product3/1 -> Atan2/2  "alongTrackDist"
  Atan2/1 -> Abs/1  "AB_to_BP_bearing"
  Compare To Constant1/1 -> out/1
  vector_AB_unit/1 -> Dot Product3/2, Cross Product/2
  vector_B_to_P_unit/1 -> Dot Product3/1, Cross Product/1

== system fw_pos_control/FW Control/fixed_wing.position_control.mode_action.l1_navigate_waypoints/If Action Subsystem ==
  vector_A_to_airplane : Inport
  ground_speed_3d : Inport  Port=2
  Action Port : ActionPort  ActionPortLabel=if(u1)
  Atan : Trigonometry  Operator=atan2
  Atan1 : Trigonometry  Operator=atan2
  Bus Creator : BusCreator  Inputs=2
  Divide : Product  Inputs=*/
  Dot Product : DotProduct  InputSameDT=on  OutDataTypeStr=Inherit: Inherit via internal rule
  Dot Product1 : DotProduct  InputSameDT=on  OutDataTypeStr=Inherit: Inherit via internal rule
  Product : Product
  Selector : Selector  InputPortWidth=3  IndexOptions=Index vector (dialog)  Indices=[3]  OutputSizes=1
  Selector1 : Selector  InputPortWidth=3  IndexOptions=Index vector (dialog)  Indices=[2]  OutputSizes=1
  Selector2 : Selector  InputPortWidth=3  IndexOptions=Index vector (dialog)  Indices=[1]  OutputSizes=1
  Sqrt : Sqrt  SaturateOnIntegerOverflow=on
  Unary Minus : UnaryMinus
  eta_bearing : Outport
  wires:
  vector_A_to_airplane/1 -> Dot Product/1, Dot Product/2, Divide/1
  Dot Product/1 -> Sqrt/1
  Sqrt/1 -> Divide/2
  Divide/1 -> Unary Minus/1, Product/1  "vector_A_to_airplane_unit"
  ground_speed_3d/1 -> Product/2, Dot Product1/1
  Product/1 -> Selector/1
  Selector/1 -> Atan/1  "xtrack_vel"
  Unary Minus/1 -> Selector1/1, Selector2/1, Dot Product1/2
  Dot Product1/1 -> Atan/2  "ltrack_vel"
  Selector2/1 -> Atan1/2
  Selector1/1 -> Atan1/1
  Atan1/1 -> Bus Creator/2  "bearing"
  Atan/1 -> Bus Creator/1  "eta"
  Bus Creator/1 -> eta_bearing/1

== system fw_pos_control/FW Control/fixed_wing.position_control.mode_action.l1_navigate_waypoints/If Action Subsystem1 ==
  vector_B_to_P_unit : Inport
  ground_speed_3d : Inport  Port=2
  Action Port : ActionPort  ActionPortLabel=elseif(u2)
  Atan : Trigonometry  Operator=atan2
  Atan1 : Trigonometry  Operator=atan2
  Bus Creator : BusCreator  Inputs=2
  Dot Product1 : DotProduct  InputSameDT=on  OutDataTypeStr=Inherit: Inherit via internal rule
  Product : Product
  Selector : Selector  InputPortWidth=3  IndexOptions=Index vector (dialog)  Indices=[3]  OutputSizes=1
  Selector1 : Selector  InputPortWidth=3  IndexOptions=Index vector (dialog)  Indices=[2]  OutputSizes=1
  Selector2 : Selector  InputPortWidth=3  IndexOptions=Index vector (dialog)  Indices=[1]  OutputSizes=1
  Unary Minus : UnaryMinus
  Unary Minus1 : UnaryMinus
  eta_bearing : Outport
  wires:
  Selector1/1 -> Atan1/1
  Selector2/1 -> Atan1/2
  Dot Product1/1 -> Atan/2  "ltrack_vel"
  Unary Minus/1 -> Dot Product1/2
  Selector/1 -> Atan/1  "xtrack_vel"
  Product/1 -> Selector/1
  ground_speed_3d/1 -> Dot Product1/1, Product/2
  vector_B_to_P_unit/1 -> Unary Minus/1, Product/1, Unary Minus1/1
  Unary Minus1/1 -> Selector1/1, Selector2/1
  Atan1/1 -> Bus Creator/2  "bearing"
  Bus Creator/1 -> eta_bearing/1
  Atan/1 -> Bus Creator/1  "eta"

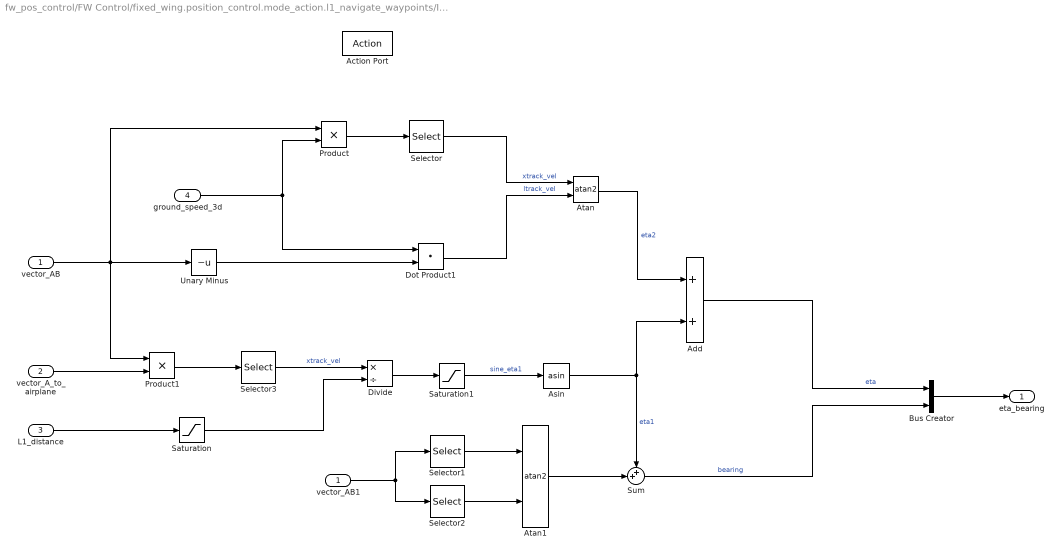
== system fw_pos_control/FW Control/fixed_wing.position_control.mode_action.l1_navigate_waypoints/If Action Subsystem2 ==
  vector_AB : Inport
  vector_A_to_airplane : Inport  Port=2
  L1_distance : Inport  Port=3
  ground_speed_3d : Inport  Port=4
  Action Port : ActionPort  ActionPortLabel=else
  Add : Sum
  Asin : Trigonometry  Operator=asin
  Atan : Trigonometry  Operator=atan2
  Atan1 : Trigonometry  Operator=atan2
  Bus Creator : BusCreator  Inputs=2
  Divide : Product  Inputs=*/
  Dot Product1 : DotProduct  InputSameDT=on  OutDataTypeStr=Inherit: Inherit via internal rule
  Product : Product
  Product1 : Product
  Saturation : Saturate  UpperLimit=single(0.1)  LowerLimit=single(-inf)
      settings: AttributesFormatString=[%<LowerLimit>,%<UpperLimit>]
  Saturation1 : Saturate  UpperLimit=single(pi/4)  LowerLimit=single(-pi/4)
      settings: AttributesFormatString=[%<LowerLimit>,%<UpperLimit>]
  Selector : Selector  InputPortWidth=3  IndexOptions=Index vector (dialog)  Indices=[3]  OutputSizes=1
  Selector1 : Selector  InputPortWidth=3  IndexOptions=Index vector (dialog)  Indices=[2]  OutputSizes=1
  Selector2 : Selector  InputPortWidth=3  IndexOptions=Index vector (dialog)  Indices=[1]  OutputSizes=1
  Selector3 : Selector  InputPortWidth=3  IndexOptions=Index vector (dialog)  Indices=[3]  OutputSizes=1
  Sum : Sum  Inputs=++|
  Unary Minus : UnaryMinus
  vector_AB1 : InportShadow
  eta_bearing : Outport
  wires:
  vector_AB/1 -> Product/1, Product1/1, Unary Minus/1
  ground_speed_3d/1 -> Product/2, Dot Product1/1
  Product/1 -> Selector/1
  Selector/1 -> Atan/1  "xtrack_vel"
  Unary Minus/1 -> Dot Product1/2
  Dot Product1/1 -> Atan/2  "ltrack_vel"
  Atan/1 -> Add/1  "eta2"
  vector_A_to_airplane/1 -> Product1/2
  L1_distance/1 -> Saturation/1
  Saturation/1 -> Divide/2
  Divide/1 -> Saturation1/1
  Saturation1/1 -> Asin/1  "sine_eta1"
  Asin/1 -> Add/2, Sum/1  "eta1"
  Selector2/1 -> Atan1/2
  vector_AB1/1 -> Selector2/1, Selector1/1
  Atan1/1 -> Sum/2
  Selector1/1 -> Atan1/1
  Product1/1 -> Selector3/1
  Selector3/1 -> Divide/1  "xtrack_vel"
  Bus Creator/1 -> eta_bearing/1
  Sum/1 -> Bus Creator/2  "bearing"
  Add/1 -> Bus Creator/1  "eta"

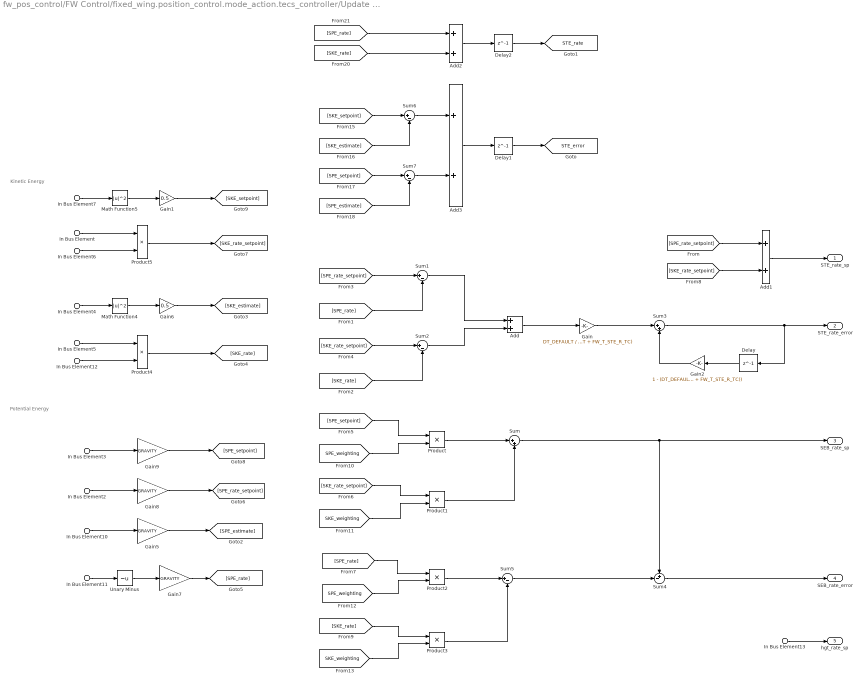
== system fw_pos_control/FW Control/fixed_wing.position_control.mode_action.tecs_controller/Update Energy Estimates ==
  note: Kinetic Energy
  note: Potential Energy
  In Bus Element11 : Inport  PortName=tecs  Element=local_pos_vz
  In Bus Element12 : Inport  PortName=tecs  Element=tas_rate_filtered
  In Bus Element : Inport  Port=2  PortName=tas_state  Element=tas
  In Bus Element4 : Inport  Port=2  PortName=tas_state  Element=tas
  In Bus Element5 : Inport  Port=2  PortName=tas_state  Element=tas
  In Bus Element6 : Inport  Port=3  PortName=tas_sp_state  Element=tas_rate_sp
  In Bus Element7 : Inport  Port=3  PortName=tas_sp_state  Element=tas_sp
  In Bus Element10 : Inport  Port=4  PortName=hgt_state  Element=hgt_sp
  In Bus Element2 : Inport  Port=5  PortName=hgt_sp_state  Element=hgt_rate_sp
  In Bus Element13 : Inport  Port=5  PortName=hgt_sp_state  Element=hgt_rate_sp
  In Bus Element3 : Inport  Port=5  PortName=hgt_sp_state  Element=hgt_sp
  Add{,1..3} (4 alike) : Sum
  Delay : Delay  DelayLength=1
  Delay1 : Delay  DelayLength=1
  Delay2 : Delay  DelayLength=1
  Gain : Gain  Gain=DT_DEFAULT / (DT_DEFAULT + FW_T_STE_R_TC)
      settings: AttributesFormatString=%<Gain>
  Gain1 : Gain  Gain=0.5  OutDataTypeStr=single
  Gain2 : Gain  Gain=1 - (DT_DEFAULT / (DT_DEFAULT + FW_T_STE_R_TC))
      settings: AttributesFormatString=%<Gain>
  Gain{5,7..9} (4 alike) : Gain  Gain=GRAVITY
  Gain6 : Gain  Gain=0.5  OutDataTypeStr=single
  Math Function4 : Math  Operator=magnitude^2  SaturateOnIntegerOverflow=on
  Math Function5 : Math  Operator=magnitude^2  SaturateOnIntegerOverflow=on
  Product{,1..5} (6 alike) : Product
  Sum : Sum  Inputs=|++
  Sum{1..2,5..7} (5 alike) : Sum  Inputs=|+-
  Sum3 : Sum  Inputs=|++
  Sum4 : Sum  Inputs=+-|
  Unary Minus : UnaryMinus
  STE_rate_sp : Outport
  STE_rate_error : Outport  Port=2
  SEB_rate_sp : Outport  Port=3
  SEB_rate_error : Outport  Port=4
  hgt_rate_sp : Outport  Port=5
  tag scope: STE_error=global, STE_rate=global
  wires:
  Math Function5/1 -> Gain1/1
  Gain9/1 -> [SPE_setpoint]
  Gain1/1 -> [SKE_setpoint]
  In Bus Element7/1 -> Math Function5/1
  In Bus Element6/1 -> Product5/2
  In Bus Element/1 -> Product5/1
  Product5/1 -> [SKE_rate_setpoint]
  Gain8/1 -> [SPE_rate_setpoint]
  In Bus Element5/1 -> Product4/1
  Gain7/1 -> [SPE_rate]
  In Bus Element10/1 -> Gain5/1
  In Bus Element3/1 -> Gain9/1
  In Bus Element2/1 -> Gain8/1
  In Bus Element12/1 -> Product4/2
  Gain5/1 -> [SPE_estimate]
  Product4/1 -> [SKE_rate]
  In Bus Element4/1 -> Math Function4/1
  Math Function4/1 -> Gain6/1
  Gain6/1 -> [SKE_estimate]
  In Bus Element11/1 -> Unary Minus/1
  [SPE_rate_setpoint] -> Sum1/1
  [SPE_rate] -> Sum1/2
  [SKE_rate_setpoint] -> Sum2/1
  [SKE_rate] -> Sum2/2
  Sum1/1 -> Add/1
  Sum2/1 -> Add/2
  Add/1 -> Gain/1
  Delay/1 -> Gain2/1
  Sum3/1 -> Delay/1, STE_rate_error/1
  Gain/1 -> Sum3/1
  Gain2/1 -> Sum3/2
  Add1/1 -> STE_rate_sp/1
  [SPE_rate_setpoint] -> Add1/1
  [SKE_rate_setpoint] -> Add1/2
  [SPE_weighting] -> Product/2
  [SPE_setpoint] -> Product/1
  [SKE_rate_setpoint] -> Product1/1
  [SKE_weighting] -> Product1/2
  Product/1 -> Sum/1
  Product1/1 -> Sum/2
  Sum/1 -> Sum4/1, SEB_rate_sp/1
  Sum4/1 -> SEB_rate_error/1
  [SPE_rate] -> Product2/1
  [SPE_weighting] -> Product2/2
  [SKE_rate] -> Product3/1
  [SKE_weighting] -> Product3/2
  Product2/1 -> Sum5/1
  Product3/1 -> Sum5/2
  Sum5/1 -> Sum4/2
  [SPE_setpoint] -> Sum7/1
  [SKE_setpoint] -> Sum6/1
  [SKE_estimate] -> Sum6/2
  [SPE_estimate] -> Sum7/2
  Sum7/1 -> Add3/2
  Sum6/1 -> Add3/1
  Add3/1 -> Delay1/1
  Delay1/1 -> [STE_error]
  [SKE_rate] -> Add2/2
  [SPE_rate] -> Add2/1
  Add2/1 -> Delay2/1
  Delay2/1 -> [STE_rate]
  Unary Minus/1 -> Gain7/1
  In Bus Element13/1 -> hgt_rate_sp/1

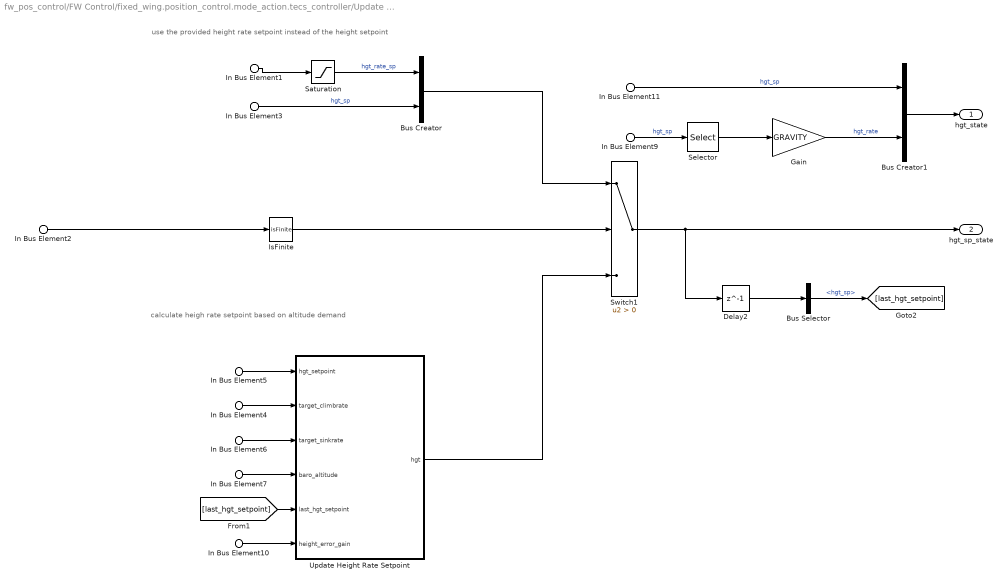
== system fw_pos_control/FW Control/fixed_wing.position_control.mode_action.tecs_controller/Update Height State and Height Setpoint State ==
  note: calculate heigh rate setpoint based on altitude demand
  note: use the provided height rate setpoint instead of the height setpoint
  In Bus Element2 : Inport  PortName=tecs  Element=hgt_rate_sp
  In Bus Element1 : Inport  PortName=tecs  Element=hgt_rate_sp
  In Bus Element7 : Inport  PortName=tecs  Element=baro_altitude
  In Bus Element3 : Inport  PortName=tecs  Element=baro_altitude
  In Bus Element11 : Inport  PortName=tecs  Element=baro_altitude
  In Bus Element4 : Inport  PortName=tecs  Element=target_climbrate
  In Bus Element5 : Inport  PortName=tecs  Element=hgt_setpoint
  In Bus Element6 : Inport  PortName=tecs  Element=target_sinkrate
  In Bus Element9 : Inport  PortName=tecs  Element=body_vel
  In Bus Element10 : Inport  PortName=tecs  Element=height_error_gain
  Bus Creator : BusCreator  Inputs=2
  Bus Creator1 : BusCreator  Inputs=2
  Bus Selector : BusSelector  OutputSignals=hgt_sp
  Delay2 : Delay  DelayLength=1
  Gain : Gain  Gain=GRAVITY
  IsFinite : RelationalOperator  Operator=isFinite  OutDataTypeStr=boolean  RndMeth=Simplest
  Saturation : Saturate  UpperLimit=FW_T_CLMB_MAX  LowerLimit=-FW_T_SINK_MAX
      settings: AttributesFormatString=[%<LowerLimit>,%<UpperLimit>]
  Selector : Selector  InputPortWidth=3  IndexOptions=Index vector (dialog)  Indices=[3]  OutputSizes=1
  Switch1 : Switch  Criteria=u2 > Threshold
  Update Height Rate Setpoint : Subsystem
  hgt_state : Outport
  hgt_sp_state : Outport  Port=2
  wires:
  Switch1/1 -> Delay2/1, hgt_sp_state/1
  Gain/1 -> Bus Creator1/2  "hgt_rate"
  Bus Creator1/1 -> hgt_state/1
  In Bus Element11/1 -> Bus Creator1/1  "hgt_sp"
  In Bus Element1/1 -> Saturation/1
  Saturation/1 -> Bus Creator/1  "hgt_rate_sp"
  Update Height Rate Setpoint/1(hgt) -> Switch1/3
  Bus Creator/1 -> Switch1/1
  IsFinite/1 -> Switch1/2
  In Bus Element2/1 -> IsFinite/1
  In Bus Element3/1 -> Bus Creator/2  "hgt_sp"
  In Bus Element5/1 -> Update Height Rate Setpoint/1(hgt_setpoint)
  In Bus Element4/1 -> Update Height Rate Setpoint/2(target_climbrate)
  In Bus Element6/1 -> Update Height Rate Setpoint/3(target_sinkrate)
  In Bus Element7/1 -> Update Height Rate Setpoint/4(baro_altitude)
  [last_hgt_setpoint] -> Update Height Rate Setpoint/5(last_hgt_setpoint)
  In Bus Element10/1 -> Update Height Rate Setpoint/6(height_error_gain)
  Delay2/1 -> Bus Selector/1
  Bus Selector/1 -> [last_hgt_setpoint]  "<hgt_sp>"
  In Bus Element9/1 -> Selector/1  "hgt_sp"
  Selector/1 -> Gain/1

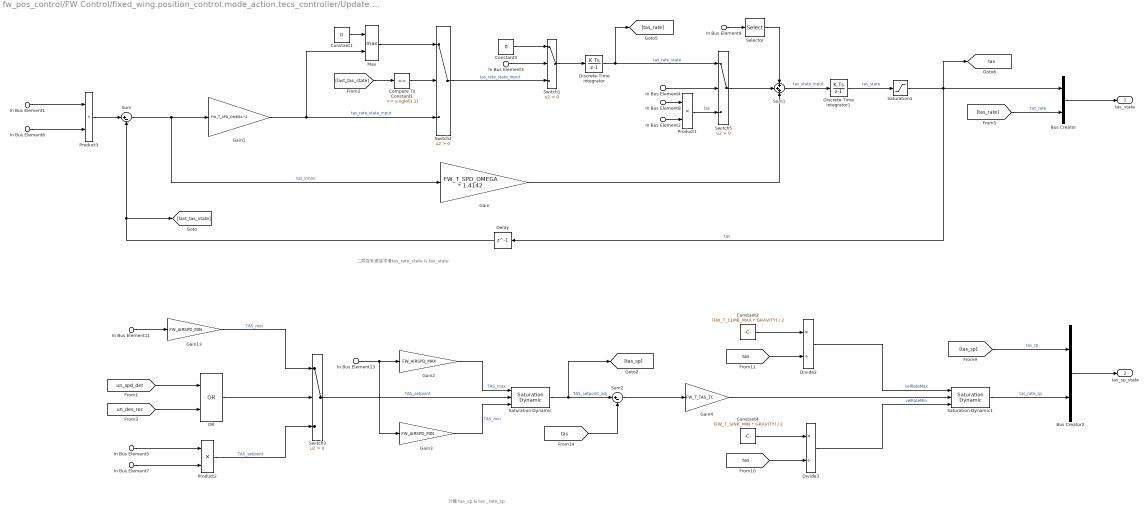
== system fw_pos_control/FW Control/fixed_wing.position_control.mode_action.tecs_controller/Update Speed State and Speed Setpoint State ==
  note: 二阶互补滤波平滑tas_rate_state & tas_state
  note: 计算 tas_sp & tas _rate_sp
  In Bus Element{2..3,6..7,11,13} (6 alike) : Inport  PortName=tecs  Element=eas_to_tas
  In Bus Element1 : Inport  PortName=tecs  Element=equivalent_airspeed
  In Bus Element5 : Inport  PortName=tecs  Element=equivalent_airspeed
  In Bus Element8 : Inport  PortName=tecs  Element=equivalent_airspeed
  In Bus Element4 : Inport  PortName=tecs  Element=in_air
  In Bus Element9 : Inport  PortName=tecs  Element=body_vel
  Bus Creator : BusCreator  Inputs=2
  Bus Creator2 : BusCreator  Inputs=2
  Compare To Constant1 : simulink/Logic and Bit Operations/Compare To Constant  relop=<=  const=single(3.1)  OutDataTypeStr=boolean
  Constant1 : Constant  Value=0  OutDataTypeStr=single
  Constant2 : Constant  Value=(FW_T_CLMB_MAX * GRAVITY) / 2
      settings: AttributesFormatString=%<Value>
  Constant3 : Constant  Value=0  OutDataTypeStr=single
  Constant4 : Constant  Value=(FW_T_SINK_MIN * GRAVITY) / 2
      settings: AttributesFormatString=%<Value>
  Delay : Delay  DelayLength=1
  Discrete-Time Integrator : DiscreteIntegrator  SampleTime=-1  ICPrevOutput=DiscIntNeverNeededParam  ICPrevScaledInput=DiscIntNeverNeededParam
  Discrete-Time Integrator1 : DiscreteIntegrator  SampleTime=-1  ICPrevOutput=DiscIntNeverNeededParam  ICPrevScaledInput=DiscIntNeverNeededParam
  Divide2 : Product  Inputs=*/
  Divide3 : Product  Inputs=*/
  Gain : Gain  Gain=FW_T_SPD_OMEGA * 1.4142
  Gain1 : Gain  Gain=FW_T_SPD_OMEGA^2  OutDataTypeStr=single
  Gain13 : Gain  Gain=FW_AIRSPD_MIN
  Gain2 : Gain  Gain=FW_AIRSPD_MAX
  Gain3 : Gain  Gain=FW_AIRSPD_MIN
  Gain4 : Gain  Gain=FW_T_TAS_TC
  Max : MinMax  Function=max  Inputs=2
  OR : Logic  Operator=OR  IconShape=distinctive  AllPortsSameDT=off  OutDataTypeStr=boolean
  Product1 : Product
  Product2 : Product
  Product3 : Product
  Saturation Dynamic : simulink/Discontinuities/Saturation Dynamic  OutMin=[]  OutMax=[]  OutDataTypeStr=Inherit: Same as second input  OutDataType=fixdt(1, 16)  OutScaling=2^-10  DoSatur=off
  Saturation Dynamic1 : simulink/Discontinuities/Saturation Dynamic  OutMin=[]  OutMax=[]  OutDataTypeStr=Inherit: Same as second input  OutDataType=fixdt(1, 16)  OutScaling=2^-10  DoSatur=off
  Saturation1 : Saturate  UpperLimit=inf  LowerLimit=3
      settings: AttributesFormatString=[%<LowerLimit>,%<UpperLimit>]
  Selector : Selector  InputPortWidth=3  IndexOptions=Index vector (dialog)  Indices=[1]  OutputSizes=1
  Sum : Sum  Inputs=|+-
  Sum1 : Sum  Inputs=+++
  Sum2 : Sum  Inputs=|+-
  Switch{1..3,5} (4 alike) : Switch  Criteria=u2 > Threshold
  tas_state : Outport
  tas_sp_state : Outport  Port=2
  tag scope: tas=global
  wires:
  In Bus Element8/1 -> Product1/1
  In Bus Element2/1 -> Product1/2
  In Bus Element1/1 -> Product3/1
  In Bus Element6/1 -> Product3/2
  Selector/1 -> Sum1/1
  Saturation Dynamic1/1 -> Bus Creator2/2  "tas_rate_sp"
  [tas_sp] -> Bus Creator2/1  "tas_sp"
  Bus Creator2/1 -> tas_sp_state/1
  [tas_rate] -> Bus Creator/2  "tas_rate"
  Bus Creator/1 -> tas_state/1
  Saturation Dynamic/1 -> Sum2/1, [tas_sp]  "TAS_setpoint_adj"
  Gain4/1 -> Saturation Dynamic1/2
  [tas] -> Divide2/2
  In Bus Element5/1 -> Product2/1
  [tas] -> Sum2/2
  Gain13/1 -> Switch3/1  "TAS_min"
  In Bus Element7/1 -> Product2/2
  [un_des_rec] -> OR/2
  Gain2/1 -> Saturation Dynamic/1  "TAS_max"
  In Bus Element11/1 -> Gain13/1
  Sum2/1 -> Gain4/1
  OR/1 -> Switch3/2
  Product2/1 -> Switch3/3  "TAS_setpoint"
  [un_spd_det] -> OR/1
  In Bus Element13/1 -> Gain3/1, Gain2/1
  Switch3/1 -> Saturation Dynamic/2  "TAS_setpoint"
  Gain3/1 -> Saturation Dynamic/3  "TAS_min"
  Divide2/1 -> Saturation Dynamic1/1  "velRateMax"
  Divide3/1 -> Saturation Dynamic1/3  "velRateMin"
  Constant4/1 -> Divide3/1
  [tas] -> Divide3/2
  Constant2/1 -> Divide2/1
  Product1/1 -> Switch5/3  "tas"
  Discrete-Time Integrator/1 -> [tas_rate], Switch5/1  "tas_rate_state"
  Switch2/1 -> Switch1/3  "tas_rate_state_input"
  Constant3/1 -> Switch1/1
  Switch5/1 -> Sum1/2
  In Bus Element4/1 -> Switch5/2
  Switch1/1 -> Discrete-Time Integrator/1
  In Bus Element3/1 -> Switch1/2
  [last_tas_state] -> Compare To Constant1/1
  Saturation1/1 -> Bus Creator/1, Delay/1, [tas]  "tas"
  Delay/1 -> [last_tas_state], Sum/2
  Max/1 -> Switch2/1
  Constant1/1 -> Max/1
  Compare To Constant1/1 -> Switch2/2
  Gain1/1 -> Switch2/3, Max/2  "tas_rate_state_input"
  Gain/1 -> Sum1/3
  Sum1/1 -> Discrete-Time Integrator1/1  "tas_state_input"
  Discrete-Time Integrator1/1 -> Saturation1/1  "tas_state"
  Sum/1 -> Gain/1, Gain1/1  "tas_innov"
  Product3/1 -> Sum/1
  In Bus Element9/1 -> Selector/1
